simulink model "Test_World_1_cs"  (R2019a)
settings: Solver=FixedStepDiscrete  StartTime=0.0  StopTime=15  FixedStep=1/300  RelTol=1e-3
PreLoadFcn:
  | mbxruntime.callbacks.PreLoadFcn(bdroot);
  | check_NUTS_defined
  | model_closed = 0;
  | assignin('base',['model_closed_' bdroot],false);
PostLoadFcn:
  | mbxruntime.callbacks.PostLoadFcn(bdroot);
InitFcn:
  | mbxruntime.callbacks.InitFcn(bdroot);
StartFcn:
  | mbxruntime.callbacks.StartFcn(bdroot);
StopFcn:
  | mbxruntime.callbacks.StopFcn(bdroot);;
  | 
model workspace: external: MAT-File .\Test_World_1_cs_hws.mat (data not in the file)
undefined symbols (not defined in the file or in its folder): AngularVelocity, Clock_, Data, Data_SL_Info, DiscIntNeverNeededParam, Encoding, Encoding_SL_Info, Header, Height, InitImageOutputDir, LinearAcceleration, Orientation, Pose, Poses, Poses_SL_Info, Position, Step, Twist, Width
libraries: robotlib x26, simulink_extras x19, PreScanSimulinkLibrary x6, PBCSimulinkLibrary x5, dspindex x4, robotcorelib x2, sharedtransform x2, visionconversions x1, visionsinks x1
(part 3 of 5)

== system Test_World_1_cs/PointCloudSensor_3 ==
  Sensor : S-Function  FunctionName=sfun_PCS  Parameters=sensorID, dataWidth, dataHeight, numChannels, dataType, timestep  SFunctionDeploymentMode=off  EnableBusSupport=off  mask(PreScan Source Block: Point Cloud Sensor){sensorID=9054, dataWidth=16, dataHeight=900, numChannels=4, dataType=0, timestep=1/20}
      mask prompts: sensorID "Sensor ID"; dataWidth "Data Width"; dataHeight "Data Height"; numChannels "Channel Count"; dataType "Data Type"; timestep "MATLAB timestep:"
      mask help: The Point Cloud Sensor provides XYZ positions relative to the sensor
      mask Help: eval('openHelp(6400)')
      mask Display: image(imread('PointCloudSensorSL.png'))
  PointCloudSensor_3 : Outport  Tag=outport/PointCloudInport  OutDataTypeStr=single  SampleTime=1/20
  wires:
  Sensor/1 -> PointCloudSensor_3/1

== system Test_World_1_cs/PointCloudSensor_4 ==
  Sensor : S-Function  FunctionName=sfun_PCS  Parameters=sensorID, dataWidth, dataHeight, numChannels, dataType, timestep  SFunctionDeploymentMode=off  EnableBusSupport=off  mask(PreScan Source Block: Point Cloud Sensor){sensorID=9055, dataWidth=16, dataHeight=900, numChannels=4, dataType=0, timestep=1/20}
      mask prompts: sensorID "Sensor ID"; dataWidth "Data Width"; dataHeight "Data Height"; numChannels "Channel Count"; dataType "Data Type"; timestep "MATLAB timestep:"
      mask help: The Point Cloud Sensor provides XYZ positions relative to the sensor
      mask Help: eval('openHelp(6400)')
      mask Display: image(imread('PointCloudSensorSL.png'))
  PointCloudSensor_4 : Outport  Tag=outport/PointCloudInport  OutDataTypeStr=single  SampleTime=1/20
  wires:
  Sensor/1 -> PointCloudSensor_4/1

== system Test_World_1_cs/PreScanTerminator ==
  Terminator : Terminator
  sfun_Terminator : S-Function  FunctionName=sfun_Terminator  Parameters=SampleTime  SFunctionDeploymentMode=off  EnableBusSupport=off  mask(Legacy Function){SFunctionSpec=void prescan_terminator_outputFcn(void ** work1, PRESCAN_TERMINATORDATA y1[1]), SampleTime=TimeStep, ShowSpec=on}
      mask prompts: SampleTime "Sample time (-1 for inherited):"; ShowSpec "Display function specification"
      mask help:
      | This block allows you to call the legacy functions specified by the following Legacy Code Tool definition:
      | def.SFunctionName = 'sfun_Terminator';
      | def.OutputFcnSpec = 'void prescan_terminator_outputFcn(void ** work1, PRESCAN_TERMINATORDATA y1[1])';
      | def.StartFcnSpec = 'void prescan_terminator_startFcn(void ** work1)';
      | def.TerminateFcnSpec = 'void prescan_terminator_terminateFcn(void ** work1)';
      | def.HeaderFiles = {'prescan_terminator_data.h'};
      | def.HostLibFiles = {'sensorinterfaced.lib'};
      | def.IncPaths = {'src', 'C:\prescandev\vislibrary\vis\..\pimp\include\sensors\InterfaceRTW'};
      | def.SrcPaths = {'src'};
      | def.LibPaths = {'C:\\prescandev\\vislibrary_build\lib'};
      | def.SampleTime = 'parameterized';
      | def.Options.language = 'C';
      mask Help: <p>This block was generated automatically by the Legacy Code Tool. For detailed help on this tool, call<a href="matlab:legacy_code('help')"> legacy_code('help')</a>.</p>
      mask Callback ShowSpec:
      | if strcmp(get_param(gcbh, 'ShowSpec'), 'on')
      |   set_param(gcbh, 'MaskDisplay', sprintf('fprintf(''%s'');', get_param(gcbh, 'SFunctionSpec')));
      | else
      |   set_param(gcbh, 'MaskDisplay', sprintf('fprintf(''%s'');', get_param(gcbh, 'FunctionName')));
      | end
      mask Display: fprintf('void prescan_terminator_outputFcn(void ** work1, PRESCAN_TERMINATORDATA y1[1])');
  wires:
  sfun_Terminator/1 -> Terminator/1

== system Test_World_1_cs/SELF_BMW_X5_SUV_1 ==
  Sensor : S-Function  FunctionName=sfun_SelfSensor  Parameters=UniqueID, TimeStep  SFunctionDeploymentMode=off  EnableBusSupport=off  mask(PreScan Source Block: SELF){UniqueID=9040, TimeStep=1/300}
      mask prompts: UniqueID "Auto-Assigned: Unique ID"; TimeStep "Auto-Assigned: Upload Period [s]"
      mask help:
      | The SELF port shows (state) information of the actor itself. The outputs are position in the experiment's axis system and the GPS coordinates, and the object's absolute velocity and compass heading.
      |
      | For more information, please click Help.
      mask Help: eval('openHelp(462)')
      mask Display: image(imread('GPS.png'))
  SELF_BMW_X5_SUV_1 : Outport  Tag=outport/SelfPort  OutDataTypeStr=Bus: PRESCAN_SELFSENSORDATA  PortDimensions=1  SampleTime=1/300
  wires:
  Sensor/1 -> SELF_BMW_X5_SUV_1/1

== system Test_World_1_cs/SELF_Citroen_C3_Hatchback_1 ==
  Sensor : S-Function  FunctionName=sfun_SelfSensor  Parameters=UniqueID, TimeStep  SFunctionDeploymentMode=off  EnableBusSupport=off  mask(PreScan Source Block: SELF){UniqueID=4877, TimeStep=1/300}
      mask prompts: UniqueID "Auto-Assigned: Unique ID"; TimeStep "Auto-Assigned: Upload Period [s]"
      mask help:
      | The SELF port shows (state) information of the actor itself. The outputs are position in the experiment's axis system and the GPS coordinates, and the object's absolute velocity and compass heading.
      |
      | For more information, please click Help.
      mask Help: eval('openHelp(462)')
      mask Display: image(imread('GPS.png'))
  SELF_Citroen_C3_Hatchback_1 : Outport  Tag=outport/SelfPort  OutDataTypeStr=Bus: PRESCAN_SELFSENSORDATA  PortDimensions=1  SampleTime=1/300
  wires:
  Sensor/1 -> SELF_Citroen_C3_Hatchback_1/1

== system Test_World_1_cs/SELF_Ford_Fiesta_Hatchback_1 ==
  Sensor : S-Function  FunctionName=sfun_SelfSensor  Parameters=UniqueID, TimeStep  SFunctionDeploymentMode=off  EnableBusSupport=off  mask(PreScan Source Block: SELF){UniqueID=4876, TimeStep=1/300}
      mask prompts: UniqueID "Auto-Assigned: Unique ID"; TimeStep "Auto-Assigned: Upload Period [s]"
      mask help:
      | The SELF port shows (state) information of the actor itself. The outputs are position in the experiment's axis system and the GPS coordinates, and the object's absolute velocity and compass heading.
      |
      | For more information, please click Help.
      mask Help: eval('openHelp(462)')
      mask Display: image(imread('GPS.png'))
  SELF_Ford_Fiesta_Hatchback_1 : Outport  Tag=outport/SelfPort  OutDataTypeStr=Bus: PRESCAN_SELFSENSORDATA  PortDimensions=1  SampleTime=1/300
  wires:
  Sensor/1 -> SELF_Ford_Fiesta_Hatchback_1/1

== system Test_World_1_cs/STATE_BMW_X5_SUV_1_bus ==
  STATE_BMW_X5_SUV_1_bus : Inport  Tag=inport/StatePort  OutDataTypeStr=Bus: PRESCAN_STATEACTUATORDATA  PortDimensions=1  SampleTime=1/300  BusOutputAsStruct=on
  Actuator : S-Function  FunctionName=sfun_StateActuator  Parameters=UniqueID, TimeStep  SFunctionDeploymentMode=off  EnableBusSupport=off  mask(PreScan Sink Block: State){UniqueID=9040, TimeStep=1/300}
      mask prompts: UniqueID "Auto-Assigned: Unique ID"; TimeStep "Auto-Assigned: Upload Period [s]"
      mask help:
      | The Actor State contains a vector signal of size (9x1), containing the following signals:
      |
      | -  Position    	(x,y,z)             	[m]
      | -  Velocity    	(vx,vy,vz)         	[m/s]
      | -  Angles       	(Roll, Pitch, Yaw)	[rad]
      |
      | The Actor state is defined in the global axis system.
      | The state is superponed on the Initial position defined in the GUI.
      |
      | For more information, please click Help.
      mask Help: eval('openHelp(222)')
      mask Display: image(imread('State.png'))
  wires:
  STATE_BMW_X5_SUV_1_bus/1 -> Actuator/1

== system Test_World_1_cs/STATE_Citroen_C3_Hatchback_1_bus ==
  STATE_Citroen_C3_Hatchback_1_bus : Inport  Tag=inport/StatePort  OutDataTypeStr=Bus: PRESCAN_STATEACTUATORDATA  PortDimensions=1  SampleTime=1/300  BusOutputAsStruct=on
  Actuator : S-Function  FunctionName=sfun_StateActuator  Parameters=UniqueID, TimeStep  SFunctionDeploymentMode=off  EnableBusSupport=off  mask(PreScan Sink Block: State){UniqueID=4877, TimeStep=1/300}
      mask prompts: UniqueID "Auto-Assigned: Unique ID"; TimeStep "Auto-Assigned: Upload Period [s]"
      mask help:
      | The Actor State contains a vector signal of size (9x1), containing the following signals:
      |
      | -  Position    	(x,y,z)             	[m]
      | -  Velocity    	(vx,vy,vz)         	[m/s]
      | -  Angles       	(Roll, Pitch, Yaw)	[rad]
      |
      | The Actor state is defined in the global axis system.
      | The state is superponed on the Initial position defined in the GUI.
      |
      | For more information, please click Help.
      mask Help: eval('openHelp(222)')
      mask Display: image(imread('State.png'))
  wires:
  STATE_Citroen_C3_Hatchback_1_bus/1 -> Actuator/1

== system Test_World_1_cs/STATE_Ford_Fiesta_Hatchback_1_bus ==
  STATE_Ford_Fiesta_Hatchback_1_bus : Inport  Tag=inport/StatePort  OutDataTypeStr=Bus: PRESCAN_STATEACTUATORDATA  PortDimensions=1  SampleTime=1/300  BusOutputAsStruct=on
  Actuator : S-Function  FunctionName=sfun_StateActuator  Parameters=UniqueID, TimeStep  SFunctionDeploymentMode=off  EnableBusSupport=off  mask(PreScan Sink Block: State){UniqueID=4876, TimeStep=1/300}
      mask prompts: UniqueID "Auto-Assigned: Unique ID"; TimeStep "Auto-Assigned: Upload Period [s]"
      mask help:
      | The Actor State contains a vector signal of size (9x1), containing the following signals:
      |
      | -  Position    	(x,y,z)             	[m]
      | -  Velocity    	(vx,vy,vz)         	[m/s]
      | -  Angles       	(Roll, Pitch, Yaw)	[rad]
      |
      | The Actor state is defined in the global axis system.
      | The state is superponed on the Initial position defined in the GUI.
      |
      | For more information, please click Help.
      mask Help: eval('openHelp(222)')
      mask Display: image(imread('State.png'))
  wires:
  STATE_Ford_Fiesta_Hatchback_1_bus/1 -> Actuator/1

== system Test_World_1_cs/Synchronizer ==
  Bus Selector1 : BusSelector  OutputSignals=FederateStopped
  Stop Simulation : Stop
  sfun_Synchronizer : S-Function  FunctionName=sfun_Synchronizer  Parameters=SampleTime  SFunctionDeploymentMode=off  EnableBusSupport=off  mask(Legacy Function){SFunctionSpec=void prescan_synchronizer_outputFcn(void ** work1, PRESCAN_SYNCHRONIZEDATA y1[1]), SampleTime=TimeStep, ShowSpec=on}
      mask prompts: SampleTime "Sample time (-1 for inherited):"; ShowSpec "Display function specification"
      mask help:
      | This block allows you to call the legacy functions specified by the following Legacy Code Tool definition:
      | def.SFunctionName = 'sfun_Synchronizer';
      | def.OutputFcnSpec = 'void prescan_synchronizer_outputFcn(void ** work1, PRESCAN_SYNCHRONIZEDATA y1[1])';
      | def.StartFcnSpec = 'void prescan_synchronizer_startFcn(void ** work1)';
      | def.TerminateFcnSpec = 'void prescan_synchronizer_terminateFcn(void ** work1)';
      | def.HeaderFiles = {'prescan_synchronizer_data.h'};
      | def.HostLibFiles = {'sensorinterfaced.lib'};
      | def.IncPaths = {'src', 'C:\prescandev\vislibrary\vis\..\pimp\include\sensors\InterfaceRTW'};
      | def.SrcPaths = {'src'};
      | def.LibPaths = {'C:\\prescandev\\vislibrary_build\lib'};
      | def.SampleTime = 'parameterized';
      | def.Options.language = 'C';
      mask Help: <p>This block was generated automatically by the Legacy Code Tool. For detailed help on this tool, call<a href="matlab:legacy_code('help')"> legacy_code('help')</a>.</p>
      mask Callback ShowSpec:
      | if strcmp(get_param(gcbh, 'ShowSpec'), 'on')
      |   set_param(gcbh, 'MaskDisplay', sprintf('fprintf(''%s'');', get_param(gcbh, 'SFunctionSpec')));
      | else
      |   set_param(gcbh, 'MaskDisplay', sprintf('fprintf(''%s'');', get_param(gcbh, 'FunctionName')));
      | end
      mask Display: fprintf('void prescan_synchronizer_outputFcn(void ** work1, PRESCAN_SYNCHRONIZEDATA y1[1])');
  wires:
  Bus Selector1/1 -> Stop Simulation/1  "<FederateStopped>"
  sfun_Synchronizer/1 -> Bus Selector1/1

== system Test_World_1_cs/camera ==
  Sensor : S-Function  FunctionName=sfun_Camera  Parameters=sensorID, dataWidth, dataHeight, channelsPerImage, numberOfImages, timestep  SFunctionDeploymentMode=off  EnableBusSupport=off  mask(PreScan Source Block: Camera Sensor){sensorID=9056, dataWidth=720, dataHeight=2880, channelsPerImage=3, numberOfImages=1, timestep=1/20}
      mask prompts: sensorID "Sensor ID"; dataWidth "Data width"; dataHeight "Data Height"; channelsPerImage "Channels per image"; numberOfImages "Number of images"; timestep "MATLAB timestep:"
      mask help: The Camera Sensor provides a color or monochrome image.
      mask Help: eval('openHelp(457)')
      mask Display: image(imread('CameraSensor.png'))
  camera : Outport  Tag=outport/Camera/CameraSensor  OutDataTypeStr=uint8  SampleTime=1/20
  wires:
  Sensor/1 -> camera/1

== system Test_World_1_cs/pose_otheCar ==
  In1 : Inport
  Enable : EnablePort
  Add5 : Sum
  Assignment : Assignment  OutputInitialize=Specify size for each dimension in table  DiagnosticForDimensions=Warning  IndexOptions=Starting index (dialog)  Indices=1  OutputSizes=1
  Assignment2 : Assignment  OutputInitialize=Specify size for each dimension in table  DiagnosticForDimensions=Warning  IndexOptions=Starting index (dialog)  Indices=1  OutputSizes=1000
  Blank Message1 : robotlib/Blank Message  messageClass=Message  entityType=geometry_msgs/PoseArray  messageType=geometry_msgs/PoseArray  SampleTime=inf
      settings: SourceProductBaseCode=RO
  Bus Assignment3 : BusAssignment  AssignedSignals=Header.Seq,Header.FrameId,Header.FrameId_SL_Info.CurrentLength,Poses,Poses_SL_Info.CurrentLength
  Bus Selector : BusSelector  OutputSignals=Poses
  Bus Selector2 : BusSelector  OutputSignals=Header.FrameId
  Constant24 : Constant  OutDataTypeStr=uint32
  Constant25 : Constant  Value=uint8(['map'])
  Memory2 : Memory  InheritSampleTime=on
  Publish2 : robotlib/Publish  topicSource=Specify your own  topic=/pose_otherCar  messageType=geometry_msgs/PoseArray  messageQueueLength=1
      settings: SourceProductBaseCode=RO
  Width : Width  DataType=uint32
  Width5 : Width  DataType=uint32
  wires:
  Blank Message1/1 -> Bus Assignment3/1, Bus Selector2/1, Bus Selector/1
  Bus Selector2/1 -> Assignment2/1  "<FrameId>"
  Assignment2/1 -> Width5/1, Bus Assignment3/3
  Constant25/1 -> Assignment2/2
  Bus Assignment3/1 -> Publish2/1
  In1/1 -> Assignment/2
  Bus Selector/1 -> Assignment/1  "<Poses>"
  Width/1 -> Bus Assignment3/6
  Assignment/1 -> Width/1, Bus Assignment3/5
  Width5/1 -> Bus Assignment3/4
  Add5/1 -> Memory2/1, Bus Assignment3/2
  Memory2/1 -> Add5/1
  Constant24/1 -> Add5/2

== system Test_World_1_cs/tl_camera ==
  Sensor : S-Function  FunctionName=sfun_Camera  Parameters=sensorID, dataWidth, dataHeight, channelsPerImage, numberOfImages, timestep  SFunctionDeploymentMode=off  EnableBusSupport=off  mask(PreScan Source Block: Camera Sensor){sensorID=12017, dataWidth=720, dataHeight=2880, channelsPerImage=3, numberOfImages=1, timestep=1/20}
      mask prompts: sensorID "Sensor ID"; dataWidth "Data width"; dataHeight "Data Height"; channelsPerImage "Channels per image"; numberOfImages "Number of images"; timestep "MATLAB timestep:"
      mask help: The Camera Sensor provides a color or monochrome image.
      mask Help: eval('openHelp(457)')
      mask Display: image(imread('CameraSensor.png'))
  tl_camera : Outport  Tag=outport/Camera/CameraSensor  OutDataTypeStr=uint8  SampleTime=1/20
  wires:
  Sensor/1 -> tl_camera/1

== system Test_World_1_cs/BMW_X5_SUV_1/Car_Pose ==
  In1 : Inport
  In2 : Inport  Port=2
  In3 : Inport  Port=3
  In4 : Inport  Port=4
  In5 : Inport  Port=5
  In6 : Inport  Port=6
  Coordinate Transformation Conversion : robotcorelib/Coordinate Transformation Conversion  InputRepresentation=Euler Angles  InputEulerSequence=XYZ  ShowTrVecInputPort=on  OutputRepresentation=Quaternion  OutputEulerSequence=ZYX  ShowTrVecOutputPort=on  SimulateUsing=Interpreted execution
      settings: SourceProductBaseCode=RO
  Data Type Conversion : DataTypeConversion
  Data Type Conversion1 : DataTypeConversion
  Data Type Conversion2 : DataTypeConversion
  Degrees to Radians1 : simulink_extras/Transformations/Degrees to Radians
  Degrees to Radians2 : simulink_extras/Transformations/Degrees to Radians
  Degrees to Radians5 : simulink_extras/Transformations/Degrees to Radians
  Mux : Mux
  Vector Concatenate2 : Concatenate  NumInputs=3
  Out1 : Outport
  wires:
  Degrees to Radians1/1 -> Vector Concatenate2/2
  Degrees to Radians5/1 -> Vector Concatenate2/1
  Vector Concatenate2/1 -> Coordinate Transformation Conversion/1
  Degrees to Radians2/1 -> Vector Concatenate2/3
  In1/1 -> Data Type Conversion/1
  In2/1 -> Data Type Conversion1/1
  In3/1 -> Data Type Conversion2/1
  In4/1 -> Degrees to Radians5/1
  In5/1 -> Degrees to Radians1/1
  In6/1 -> Degrees to Radians2/1
  Data Type Conversion/1 -> Mux/1
  Data Type Conversion1/1 -> Mux/2
  Data Type Conversion2/1 -> Mux/3
  Coordinate Transformation Conversion/1 -> Mux/4
  Mux/1 -> Out1/1

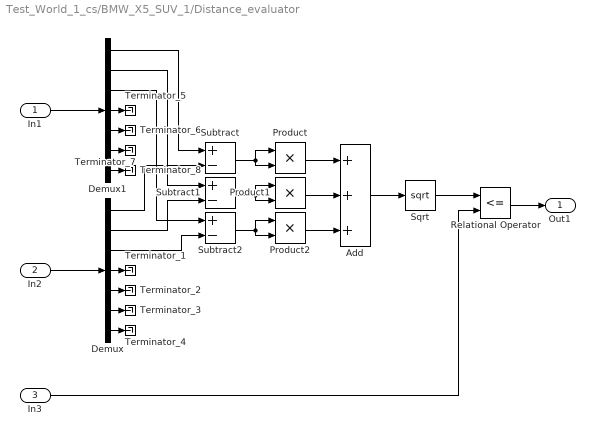
== system Test_World_1_cs/BMW_X5_SUV_1/Distance_evaluator ==
  In1 : Inport
  In2 : Inport  Port=2
  In3 : Inport  Port=3
  Add : Sum  Inputs=3
  Demux : Demux  Outputs=7
  Demux1 : Demux  Outputs=7
  Product : Product
  Product1 : Product
  Product2 : Product
  Relational Operator : RelationalOperator  Operator=<=  OutDataTypeStr=boolean  RndMeth=Simplest
  Sqrt : Sqrt  SaturateOnIntegerOverflow=on
  Subtract : Sum  Inputs=+-
  Subtract1 : Sum  Inputs=+-
  Subtract2 : Sum  Inputs=+-
  Terminator_{1..8} (8 alike) : Terminator
  Out1 : Outport
  wires:
  Relational Operator/1 -> Out1/1
  In1/1 -> Demux1/1
  In2/1 -> Demux/1
  Demux1/1 -> Subtract/1
  Demux1/2 -> Subtract1/1
  Demux1/3 -> Subtract2/1
  Demux/1 -> Subtract/2
  Demux/2 -> Subtract1/2
  Demux/3 -> Subtract2/2
  Subtract/1 -> Product/1, Product/2
  Subtract1/1 -> Product1/1, Product1/2
  Subtract2/1 -> Product2/1, Product2/2
  Product/1 -> Add/1
  Product1/1 -> Add/2
  Product2/1 -> Add/3
  Add/1 -> Sqrt/1
  Sqrt/1 -> Relational Operator/1
  In3/1 -> Relational Operator/2
  Demux/4 -> Terminator_1/1
  Demux/5 -> Terminator_2/1
  Demux/6 -> Terminator_3/1
  Demux/7 -> Terminator_4/1
  Demux1/4 -> Terminator_5/1
  Demux1/5 -> Terminator_6/1
  Demux1/6 -> Terminator_7/1
  Demux1/7 -> Terminator_8/1

== system Test_World_1_cs/BMW_X5_SUV_1/Dynamics_Empty ==
  note: For state mode 'Dynamic' positions
      | are not taken into account, as they
      | are computed by integrating velocity.
      | Click annotation for Help.
  Bus Selector : BusSelector  OutputSignals=Twist.Linear.X,Twist.Linear.Y,Twist.Linear.Z,Twist.Angular.X,Twist.Angular.Y,Twist.Angular.Z
  Data Type Conversion{,1..5} (6 alike) : DataTypeConversion
  Discrete-Time Integrator1 : DiscreteIntegrator  SampleTime=-1  ICPrevOutput=DiscIntNeverNeededParam  ICPrevScaledInput=DiscIntNeverNeededParam
  Discrete-Time Integrator2 : DiscreteIntegrator  SampleTime=-1  ICPrevOutput=DiscIntNeverNeededParam  ICPrevScaledInput=DiscIntNeverNeededParam
  Discrete-Time Integrator3 : DiscreteIntegrator  SampleTime=-1  ICPrevOutput=DiscIntNeverNeededParam  ICPrevScaledInput=DiscIntNeverNeededParam
  Ground_1 : Ground
  Ground_2 : Ground
  Ground_3 : Ground
  MuxState : Subsystem  Tag=mux/State  mask(Empty Dynamics State Block){positioningmode=off, TimeStep=1/300}
      mask prompts: positioningmode "Positioning Mode"; TimeStep "Auto Assigned: Time Step [s]"
      mask help:
      | Build the state of an actor based on user input.
      | The user can either use positioning mode or dynamics mode.
      | - When using positioning mode the position and orientation of the actor are set directly based on the input. Expected input is relative to the initial position and orientation of the actor. It's also possible to specify the velocity of the actor, though this input isn't used, only passed on.
      | - When using dynamics mode the position input is ignored. Expected input is velocity and orientation. The velocity is relative the current orientation of the actor, while orientation is relative to its initial orientation. The position of the actor is calculated based on the velocity and orientation given.
      settings: DeleteFcn=PreScanBlockDeleteFcn;
  STATE_BMW_X5_SUV_1 : Subsystem  Tag=mux/StatePort  Priority=0  LoadFcn=load PrescanStateActuatorData  mask(PreScan Sink Block: State){x0=19.2335, y0=197.6423, z0=0.69, Roll0=0, Pitch0=0, Yaw0=0.26655, TimeStep=1/300}
      mask prompts: x0 "Ini x-position VEHICLE wrt GLOBAL axis system [m]"; y0 "Ini y-position VEHICLE wrt GLOBAL axis system [m]"; z0 "Ini z-position VEHICLE wrt GLOBAL axis system [m]"; Roll0 "Ini roll-angle BODY wrt VEHICLE axis system [deg]"; Pitch0 "Ini pitch-angle BODY wrt VEHICLE axis system [deg]"; Yaw0 "Ini yaw-angle VEHICLE wrt GLOBAL axis system [deg]"; TimeStep "Auto-Assigned: Upload Period [s]"
      mask help:
      | The Actor State contains a vector signal of size (9x1), containing the following signals:
      |
      | -  Position                  (x,y,z)                                     [m]
      | -  Velocity                  (vx,vy,vz)                               [m/s]
      | -  Angles                    (Roll, Pitch, Yaw)                   [rad]
      |
      | The Actor state is defined in the global axis system.
      | The state is superponed on the Initial position defined in the GUI.
      |
      | For more information, please click Help.
      settings: DeleteFcn=PreScanBlockDeleteFcn;
      mask Help: eval('openHelp(222)')
      mask Display: image(imread('State.png'))
  Scope : Scope
  Sine Wave Function : Sin  Amplitude=0.1  SampleTime=0
  Subscribe : robotlib/Subscribe  topicSource=Select from ROS network  topic=/TwistS  messageType=geometry_msgs/TwistStamped  sampleTime=-1  messageQueueLength=1
      settings: SourceProductBaseCode=RO
  Terminator_1 : Terminator
  Terminator_2 : Terminator
  State : Outport  Tag=outport/StateOutport  SampleTime=1/300
  tag scope: x_speed=global
  wires:
  Bus Selector/1 -> Data Type Conversion/1, Scope/1  "<X>"
  Bus Selector/2 -> Data Type Conversion1/1  "<Y>"
  Bus Selector/3 -> Data Type Conversion2/1  "<Z>"
  Bus Selector/4 -> Data Type Conversion3/1  "<X>"
  Data Type Conversion3/1 -> Discrete-Time Integrator3/1
  Bus Selector/5 -> Data Type Conversion4/1  "<Y>"
  Data Type Conversion4/1 -> Discrete-Time Integrator2/1
  Bus Selector/6 -> Data Type Conversion5/1  "<Z>"
  Data Type Conversion5/1 -> Discrete-Time Integrator1/1
  Subscribe/2 -> Bus Selector/1
  Data Type Conversion/1 -> [x_speed], MuxState/4(dx [m/s])
  Data Type Conversion1/1 -> MuxState/5(dy [m/s])
  Data Type Conversion2/1 -> MuxState/6(dz [m/s])
  Discrete-Time Integrator3/1 -> MuxState/7(R [rad])
  Discrete-Time Integrator2/1 -> MuxState/8(P [rad])
  Discrete-Time Integrator1/1 -> MuxState/9(Y [rad])
  MuxState/1(state) -> STATE_BMW_X5_SUV_1/1(State)
  STATE_BMW_X5_SUV_1/1(StateBus) -> State/1
  Ground_1/1 -> MuxState/1(x [m])
  Ground_2/1 -> MuxState/2(y [m])
  Ground_3/1 -> MuxState/3(z [m])
  Sine Wave Function/1 -> Terminator_1/1
  Subscribe/1 -> Terminator_2/1

== system Test_World_1_cs/BMW_X5_SUV_1/Frequency evaluator ==
  In1 : Inport
  Add : Sum  Inputs=+-
  Clock2 : Clock
  Constant : Constant
  Divide : Product  Inputs=*/
  Memory : Memory
  Relational Operator : RelationalOperator  OutDataTypeStr=boolean  RndMeth=Simplest
  Switch : Switch  Criteria=u2 > Threshold
  Out1 : Outport
  wires:
  Memory/1 -> Switch/3, Add/2
  Switch/1 -> Memory/1
  Add/1 -> Relational Operator/1
  Relational Operator/1 -> Switch/2, Out1/1
  Clock2/1 -> Add/1, Switch/1
  In1/1 -> Divide/2
  Constant/1 -> Divide/1
  Divide/1 -> Relational Operator/2

== system Test_World_1_cs/BMW_X5_SUV_1/Frequency evaluator1 ==
  In1 : Inport
  Add : Sum  Inputs=+-
  Clock2 : Clock
  Constant : Constant
  Divide : Product  Inputs=*/
  Memory : Memory
  Relational Operator : RelationalOperator  OutDataTypeStr=boolean  RndMeth=Simplest
  Switch : Switch  Criteria=u2 > Threshold
  Out1 : Outport
  wires:
  Memory/1 -> Switch/3, Add/2
  Switch/1 -> Memory/1
  Add/1 -> Relational Operator/1
  Relational Operator/1 -> Switch/2, Out1/1
  Clock2/1 -> Add/1, Switch/1
  In1/1 -> Divide/2
  Constant/1 -> Divide/1
  Divide/1 -> Relational Operator/2

== system Test_World_1_cs/BMW_X5_SUV_1/Frequency evaluator2 ==
  In1 : Inport
  Add : Sum  Inputs=+-
  Clock2 : Clock
  Constant : Constant
  Divide : Product  Inputs=*/
  Memory : Memory
  Relational Operator : RelationalOperator  OutDataTypeStr=boolean  RndMeth=Simplest
  Switch : Switch  Criteria=u2 > Threshold
  Out1 : Outport
  wires:
  Memory/1 -> Switch/3, Add/2
  Switch/1 -> Memory/1
  Add/1 -> Relational Operator/1
  Relational Operator/1 -> Switch/2, Out1/1
  Clock2/1 -> Add/1, Switch/1
  In1/1 -> Divide/2
  Constant/1 -> Divide/1
  Divide/1 -> Relational Operator/2

== system Test_World_1_cs/BMW_X5_SUV_1/Frequency evaluator3 ==
  In1 : Inport
  Add : Sum  Inputs=+-
  Clock2 : Clock
  Constant : Constant
  Divide : Product  Inputs=*/
  Memory : Memory
  Relational Operator : RelationalOperator  OutDataTypeStr=boolean  RndMeth=Simplest
  Switch : Switch  Criteria=u2 > Threshold
  Out1 : Outport
  wires:
  Memory/1 -> Switch/3, Add/2
  Switch/1 -> Memory/1
  Add/1 -> Relational Operator/1
  Relational Operator/1 -> Switch/2, Out1/1
  Clock2/1 -> Add/1, Switch/1
  In1/1 -> Divide/2
  Constant/1 -> Divide/1
  Divide/1 -> Relational Operator/2

== system Test_World_1_cs/BMW_X5_SUV_1/Frequency evaluator4 ==
  In1 : Inport
  Add : Sum  Inputs=+-
  Clock2 : Clock
  Constant : Constant
  Divide : Product  Inputs=*/
  Memory : Memory
  Relational Operator : RelationalOperator  OutDataTypeStr=boolean  RndMeth=Simplest
  Switch : Switch  Criteria=u2 > Threshold
  Out1 : Outport
  wires:
  Memory/1 -> Switch/3, Add/2
  Switch/1 -> Memory/1
  Add/1 -> Relational Operator/1
  Relational Operator/1 -> Switch/2, Out1/1
  Clock2/1 -> Add/1, Switch/1
  In1/1 -> Divide/2
  Constant/1 -> Divide/1
  Divide/1 -> Relational Operator/2

== system Test_World_1_cs/BMW_X5_SUV_1/Frequency evaluator5 ==
  In1 : Inport
  Add : Sum  Inputs=+-
  Clock2 : Clock
  Constant : Constant
  Divide : Product  Inputs=*/
  Memory : Memory
  Relational Operator : RelationalOperator  OutDataTypeStr=boolean  RndMeth=Simplest
  Switch : Switch  Criteria=u2 > Threshold
  Out1 : Outport
  wires:
  Memory/1 -> Switch/3, Add/2
  Switch/1 -> Memory/1
  Add/1 -> Relational Operator/1
  Relational Operator/1 -> Switch/2, Out1/1
  Clock2/1 -> Add/1, Switch/1
  In1/1 -> Divide/2
  Constant/1 -> Divide/1
  Divide/1 -> Relational Operator/2

== system Test_World_1_cs/BMW_X5_SUV_1/Frequency evaluator6 ==
  In1 : Inport
  Add : Sum  Inputs=+-
  Clock2 : Clock
  Constant : Constant
  Divide : Product  Inputs=*/
  Memory : Memory
  Relational Operator : RelationalOperator  OutDataTypeStr=boolean  RndMeth=Simplest
  Switch : Switch  Criteria=u2 > Threshold
  Out1 : Outport
  wires:
  Divide/1 -> Relational Operator/2
  Constant/1 -> Divide/1
  In1/1 -> Divide/2
  Clock2/1 -> Switch/1, Add/1
  Relational Operator/1 -> Out1/1, Switch/2
  Add/1 -> Relational Operator/1
  Switch/1 -> Memory/1
  Memory/1 -> Add/2, Switch/3

== system Test_World_1_cs/BMW_X5_SUV_1/Frequency evaluator7 ==
  In1 : Inport
  Add : Sum  Inputs=+-
  Clock2 : Clock
  Constant : Constant
  Divide : Product  Inputs=*/
  Memory : Memory
  Relational Operator : RelationalOperator  OutDataTypeStr=boolean  RndMeth=Simplest
  Switch : Switch  Criteria=u2 > Threshold
  Out1 : Outport
  wires:
  Divide/1 -> Relational Operator/2
  Constant/1 -> Divide/1
  In1/1 -> Divide/2
  Clock2/1 -> Switch/1, Add/1
  Relational Operator/1 -> Out1/1, Switch/2
  Add/1 -> Relational Operator/1
  Switch/1 -> Memory/1
  Memory/1 -> Add/2, Switch/3

== system Test_World_1_cs/BMW_X5_SUV_1/HumViewCamera_CM_Demux ==
  In1 : Inport
  Selector : Selector  NumberOfDimensions=2  InputPortWidth=3  IndexOptions=Index vector (dialog),Index vector (dialog)  Indices=-1,1:hres  OutputSizes=1,1
  Selector1 : Selector  NumberOfDimensions=2  InputPortWidth=3  IndexOptions=Index vector (dialog),Index vector (dialog)  Indices=-1,hres+1:hres*2  OutputSizes=1,1
  Selector2 : Selector  NumberOfDimensions=2  InputPortWidth=3  IndexOptions=Index vector (dialog),Index vector (dialog)  Indices=-1,hres*2+1:hres*3  OutputSizes=1,1
  R : Outport
  G : Outport  Port=2
  B : Outport  Port=3
  wires:
  In1/1 -> Selector1/1, Selector/1, Selector2/1
  Selector/1 -> R/1
  Selector1/1 -> G/1
  Selector2/1 -> B/1

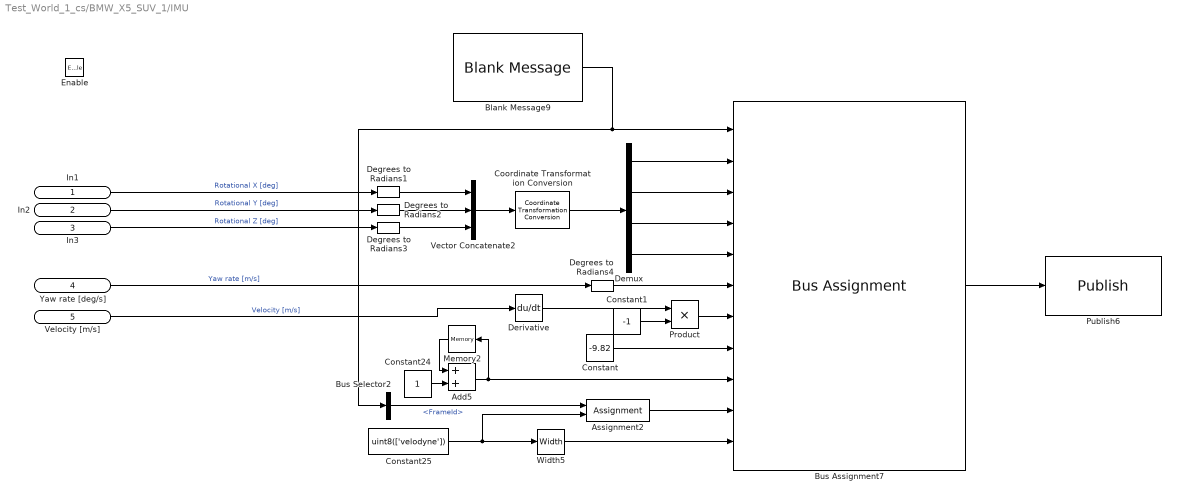
== system Test_World_1_cs/BMW_X5_SUV_1/IMU ==
  In1 : Inport
  In2 : Inport  Port=2
  In3 : Inport  Port=3
  Yaw rate [deg/s] : Inport  Port=4
  Velocity [m/s] : Inport  Port=5
  Enable : EnablePort
  Add5 : Sum
  Assignment2 : Assignment  OutputInitialize=Specify size for each dimension in table  DiagnosticForDimensions=Warning  IndexOptions=Starting index (dialog)  Indices=1  OutputSizes=1000
  Blank Message9 : robotlib/Blank Message  messageClass=Message  entityType=sensor_msgs/Imu  messageType=sensor_msgs/Imu  SampleTime=inf
      settings: SourceProductBaseCode=RO
  Bus Assignment7 : BusAssignment  AssignedSignals=Orientation.W,Orientation.X,Orientation.Y,Orientation.Z,AngularVelocity.Z,LinearAcceleration.X,LinearAcceleration.Z,Header.Seq,Header.FrameId,Header.FrameId_SL_Info.CurrentLength
  Bus Selector2 : BusSelector  OutputSignals=Header.FrameId
  Constant : Constant  Value=-9.82
  Constant1 : Constant  Value=-1
  Constant24 : Constant  OutDataTypeStr=uint32
  Constant25 : Constant  Value=uint8(['velodyne'])
  Coordinate Transformation Conversion : robotcorelib/Coordinate Transformation Conversion  InputRepresentation=Euler Angles  InputEulerSequence=XYZ  ShowTrVecInputPort=on  OutputRepresentation=Quaternion  OutputEulerSequence=ZYX  ShowTrVecOutputPort=on  SimulateUsing=Interpreted execution
      settings: SourceProductBaseCode=RO
  Degrees to Radians{1..4} (4 alike) : simulink_extras/Transformations/Degrees to Radians
  Demux : Demux
  Derivative : Derivative
  Memory2 : Memory  InheritSampleTime=on
  Product : Product
  Publish6 : robotlib/Publish  topicSource=Select from ROS network  topic=/imu_raw  messageType=sensor_msgs/Imu  messageQueueLength=1
      settings: SourceProductBaseCode=RO
  Vector Concatenate2 : Concatenate  NumInputs=3
  Width5 : Width  DataType=uint32
  wires:
  Product/1 -> Bus Assignment7/7
  Constant1/1 -> Product/2
  In3/1 -> Degrees to Radians3/1  "Rotational Z [deg]"
  In2/1 -> Degrees to Radians2/1  "Rotational Y [deg]"
  In1/1 -> Degrees to Radians1/1  "Rotational X [deg]"
  Constant/1 -> Bus Assignment7/8
  Velocity [m/s]/1 -> Derivative/1  "Velocity [m/s]"
  Yaw rate [deg/s]/1 -> Degrees to Radians4/1  "Yaw rate [m/s]"
  Demux/4 -> Bus Assignment7/5
  Demux/1 -> Bus Assignment7/2
  Coordinate Transformation Conversion/1 -> Demux/1
  Demux/3 -> Bus Assignment7/4
  Vector Concatenate2/1 -> Coordinate Transformation Conversion/1
  Degrees to Radians3/1 -> Vector Concatenate2/3
  Demux/2 -> Bus Assignment7/3
  Degrees to Radians2/1 -> Vector Concatenate2/2
  Derivative/1 -> Product/1
  Assignment2/1 -> Bus Assignment7/10
  Degrees to Radians4/1 -> Bus Assignment7/6
  Memory2/1 -> Add5/1
  Bus Assignment7/1 -> Publish6/1
  Add5/1 -> Bus Assignment7/9, Memory2/1
  Width5/1 -> Bus Assignment7/11
  Blank Message9/1 -> Bus Assignment7/1, Bus Selector2/1
  Bus Selector2/1 -> Assignment2/1  "<FrameId>"
  Constant25/1 -> Width5/1, Assignment2/2
  Constant24/1 -> Add5/2
  Degrees to Radians1/1 -> Vector Concatenate2/1

== system Test_World_1_cs/BMW_X5_SUV_1/PhysicsBasedCameraSensor_1_PBCPose_Control_Mux ==
  Position [m] : Inport
  Orientation [rad] : Inport  Port=2
  Bus Creator1 : BusCreator  Inputs=12  OutDataTypeStr=Bus: PRESCAN_PBCPOSE_DATA  NonVirtualBus=on
  Demux{,1..3} (4 alike) : Demux  Outputs=3
  SignalChanged : PBCSimulinkLibrary/SignalChanged  SystemSampleTime=-1
  SignalChanged1 : PBCSimulinkLibrary/SignalChanged  SystemSampleTime=-1
  Bus : Outport
  wires:
  Demux1/3 -> Bus Creator1/12  "OrientationYaw"
  Demux1/2 -> Bus Creator1/11  "OrientationPitch"
  Demux1/1 -> Bus Creator1/10  "OrientationRoll"
  Demux3/3 -> Bus Creator1/9  "OrientationYawDefined"
  Demux3/2 -> Bus Creator1/8  "OrientationPitchDefined"
  Demux3/1 -> Bus Creator1/7  "OrientationRollDefined"
  Demux/3 -> Bus Creator1/6  "PositionZ"
  Demux/2 -> Bus Creator1/5  "PositionY"
  Demux/1 -> Bus Creator1/4  "PositionX"
  Demux2/3 -> Bus Creator1/3  "PositionZDefined"
  Demux2/2 -> Bus Creator1/2  "PositionYDefined"
  Demux2/1 -> Bus Creator1/1  "PositionXDefined"
  SignalChanged1/1 -> Demux3/1
  SignalChanged/1 -> Demux2/1
  Bus Creator1/1 -> Bus/1
  Position [m]/1 -> SignalChanged/1, Demux/1
  Orientation [rad]/1 -> SignalChanged1/1, Demux1/1

== system Test_World_1_cs/BMW_X5_SUV_1/PhysicsBasedCameraSensor_1_PBC_Control_Mux ==
  IntegrationTime [s] : Inport
  DigitalGain [-] : Inport  Port=2
  InterRowIntegrationDelay [s] : Inport  Port=3
  AnalogGain : Constant  Value=0
  AnalogGainDefined : Constant  Value=false
  Bus Creator1 : BusCreator  Inputs=14  OutDataTypeStr=Bus: PRESCAN_PBCCONTROL_DATA  NonVirtualBus=on
  DigitalGain1 : Constant  Value=0
  DigitalGain2 : Constant  Value=0
  DigitalGain3 : Constant  Value=0
  DigitalGainDefined1 : Constant  Value=false
  DigitalGainDefined2 : Constant  Value=false
  DigitalGainDefined3 : Constant  Value=false
  NonNegativeSignalChanged1 : PBCSimulinkLibrary/NonNegativeSignalChanged  SystemSampleTime=-1
  NonNegativeSignalChanged2 : PBCSimulinkLibrary/NonNegativeSignalChanged  SystemSampleTime=-1
  NonNegativeSignalChanged7 : PBCSimulinkLibrary/NonNegativeSignalChanged  SystemSampleTime=-1
  Bus : Outport
  wires:
  NonNegativeSignalChanged7/1 -> Bus Creator1/13  "InterRowIntegrationDelayDefined"
  InterRowIntegrationDelay [s]/1 -> Bus Creator1/14, NonNegativeSignalChanged7/1  "InterRowIntegrationDelay"
  AnalogGainDefined/1 -> Bus Creator1/11  "AnalogGainDefined"
  AnalogGain/1 -> Bus Creator1/12  "AnalogGain"
  DigitalGainDefined3/1 -> Bus Creator1/9  "DigitalGain3Defined"
  DigitalGainDefined2/1 -> Bus Creator1/7  "DigitalGain2Defined"
  DigitalGainDefined1/1 -> Bus Creator1/5  "DigitalGain1Defined"
  NonNegativeSignalChanged2/1 -> Bus Creator1/3  "DigitalGain0Defined"
  NonNegativeSignalChanged1/1 -> Bus Creator1/1  "IntegrationTimeDefined"
  DigitalGain3/1 -> Bus Creator1/10  "DigitalGain3"
  DigitalGain2/1 -> Bus Creator1/8  "DigitalGain2"
  DigitalGain1/1 -> Bus Creator1/6  "DigitalGain1"
  DigitalGain [-]/1 -> Bus Creator1/4, NonNegativeSignalChanged2/1  "DigitalGain0"
  IntegrationTime [s]/1 -> Bus Creator1/2, NonNegativeSignalChanged1/1  "IntegrationTime"
  Bus Creator1/1 -> Bus/1

== system Test_World_1_cs/BMW_X5_SUV_1/PhysicsBasedCameraSensor_1_capture_opticsandsensor_Demux ==
  note: This block exists for legacy compatibility only
  In1 : Inport
  I : Outport
  wires:
  In1/1 -> I/1

== system Test_World_1_cs/BMW_X5_SUV_1/PointCloudSensor_1_Angles_Demux ==
  In2 : Inport
  Selector : Selector  NumberOfDimensions=2  InputPortWidth=3  IndexOptions=Index vector (dialog),Index vector (dialog)  Indices=-1,offset+1:(offset+hres)  OutputSizes=1,1
  Selector1 : Selector  NumberOfDimensions=2  InputPortWidth=3  IndexOptions=Index vector (dialog),Index vector (dialog)  Indices=-1,(offset+hres+1):(offset+2*hres)  OutputSizes=1,1
  Theta : Outport
  Phi : Outport  Port=2
  wires:
  Selector1/1 -> Phi/1
  Selector/1 -> Theta/1
  In2/1 -> Selector/1, Selector1/1

== system Test_World_1_cs/BMW_X5_SUV_1/PointCloudSensor_1_Intensity_Demux ==
  In1 : Inport
  Selector3 : Selector  NumberOfDimensions=2  InputPortWidth=3  IndexOptions=Index vector (dialog),Index vector (dialog)  Indices=-1,offset+1:(offset+hres)  OutputSizes=1,1
  Intensity : Outport
  wires:
  Selector3/1 -> Intensity/1
  In1/1 -> Selector3/1

== system Test_World_1_cs/BMW_X5_SUV_1/PointCloudSensor_1_Range_Demux ==
  In1 : Inport
  Selector : Selector  NumberOfDimensions=2  InputPortWidth=3  IndexOptions=Index vector (dialog),Index vector (dialog)  Indices=-1,offset+1:(offset+hres)  OutputSizes=1,1
  Range : Outport
  wires:
  Selector/1 -> Range/1
  In1/1 -> Selector/1

== system Test_World_1_cs/BMW_X5_SUV_1/PointCloudSensor_2_Angles_Demux ==
  In2 : Inport
  Selector : Selector  NumberOfDimensions=2  InputPortWidth=3  IndexOptions=Index vector (dialog),Index vector (dialog)  Indices=-1,offset+1:(offset+hres)  OutputSizes=1,1
  Selector1 : Selector  NumberOfDimensions=2  InputPortWidth=3  IndexOptions=Index vector (dialog),Index vector (dialog)  Indices=-1,(offset+hres+1):(offset+2*hres)  OutputSizes=1,1
  Theta : Outport
  Phi : Outport  Port=2
  wires:
  Selector1/1 -> Phi/1
  Selector/1 -> Theta/1
  In2/1 -> Selector/1, Selector1/1

== system Test_World_1_cs/BMW_X5_SUV_1/PointCloudSensor_2_Intensity_Demux ==
  In1 : Inport
  Selector3 : Selector  NumberOfDimensions=2  InputPortWidth=3  IndexOptions=Index vector (dialog),Index vector (dialog)  Indices=-1,offset+1:(offset+hres)  OutputSizes=1,1
  Intensity : Outport
  wires:
  Selector3/1 -> Intensity/1
  In1/1 -> Selector3/1

== system Test_World_1_cs/BMW_X5_SUV_1/PointCloudSensor_2_Range_Demux ==
  In1 : Inport
  Selector : Selector  NumberOfDimensions=2  InputPortWidth=3  IndexOptions=Index vector (dialog),Index vector (dialog)  Indices=-1,offset+1:(offset+hres)  OutputSizes=1,1
  Range : Outport
  wires:
  Selector/1 -> Range/1
  In1/1 -> Selector/1

== system Test_World_1_cs/BMW_X5_SUV_1/PointCloudSensor_3_Angles_Demux ==
  In2 : Inport
  Selector : Selector  NumberOfDimensions=2  InputPortWidth=3  IndexOptions=Index vector (dialog),Index vector (dialog)  Indices=-1,offset+1:(offset+hres)  OutputSizes=1,1
  Selector1 : Selector  NumberOfDimensions=2  InputPortWidth=3  IndexOptions=Index vector (dialog),Index vector (dialog)  Indices=-1,(offset+hres+1):(offset+2*hres)  OutputSizes=1,1
  Theta : Outport
  Phi : Outport  Port=2
  wires:
  Selector1/1 -> Phi/1
  Selector/1 -> Theta/1
  In2/1 -> Selector/1, Selector1/1

== system Test_World_1_cs/BMW_X5_SUV_1/PointCloudSensor_3_Intensity_Demux ==
  In1 : Inport
  Selector3 : Selector  NumberOfDimensions=2  InputPortWidth=3  IndexOptions=Index vector (dialog),Index vector (dialog)  Indices=-1,offset+1:(offset+hres)  OutputSizes=1,1
  Intensity : Outport
  wires:
  Selector3/1 -> Intensity/1
  In1/1 -> Selector3/1

== system Test_World_1_cs/BMW_X5_SUV_1/PointCloudSensor_3_Range_Demux ==
  In1 : Inport
  Selector : Selector  NumberOfDimensions=2  InputPortWidth=3  IndexOptions=Index vector (dialog),Index vector (dialog)  Indices=-1,offset+1:(offset+hres)  OutputSizes=1,1
  Range : Outport
  wires:
  Selector/1 -> Range/1
  In1/1 -> Selector/1

== system Test_World_1_cs/BMW_X5_SUV_1/PointCloudSensor_4_Angles_Demux ==
  In2 : Inport
  Selector : Selector  NumberOfDimensions=2  InputPortWidth=3  IndexOptions=Index vector (dialog),Index vector (dialog)  Indices=-1,offset+1:(offset+hres)  OutputSizes=1,1
  Selector1 : Selector  NumberOfDimensions=2  InputPortWidth=3  IndexOptions=Index vector (dialog),Index vector (dialog)  Indices=-1,(offset+hres+1):(offset+2*hres)  OutputSizes=1,1
  Theta : Outport
  Phi : Outport  Port=2
  wires:
  Selector1/1 -> Phi/1
  Selector/1 -> Theta/1
  In2/1 -> Selector/1, Selector1/1

== system Test_World_1_cs/BMW_X5_SUV_1/PointCloudSensor_4_Intensity_Demux ==
  In1 : Inport
  Selector3 : Selector  NumberOfDimensions=2  InputPortWidth=3  IndexOptions=Index vector (dialog),Index vector (dialog)  Indices=-1,offset+1:(offset+hres)  OutputSizes=1,1
  Intensity : Outport
  wires:
  Selector3/1 -> Intensity/1
  In1/1 -> Selector3/1

== system Test_World_1_cs/BMW_X5_SUV_1/PointCloudSensor_4_Range_Demux ==
  In1 : Inport
  Selector : Selector  NumberOfDimensions=2  InputPortWidth=3  IndexOptions=Index vector (dialog),Index vector (dialog)  Indices=-1,offset+1:(offset+hres)  OutputSizes=1,1
  Range : Outport
  wires:
  Selector/1 -> Range/1
  In1/1 -> Selector/1

== system Test_World_1_cs/BMW_X5_SUV_1/SELF_Demux ==
  SELF : Inport  OutDataTypeStr=Bus: PRESCAN_SELFSENSORDATA
  Bus Selector : BusSelector  OutputSignals=PositionX,PositionY,PositionZ,OrientationRoll,OrientationPitch,OrientationYaw,Velocity,Yaw_rate,Lat,Long,Alt
  Demux2 : Demux  Outputs=3
  Gain : Gain  Gain=180/pi
  Gain1 : Gain  Gain=180/pi
  Vector Concatenate1 : Concatenate  NumInputs=3
  compas converter : Subsystem
  x [m] : Outport
  y [m] : Outport  Port=2
  z [m] : Outport  Port=3
  rotx [deg] : Outport  Port=4
  roty [deg] : Outport  Port=5
  rotz [deg] : Outport  Port=6
  GPS lat [deg] : Outport  Port=7
  GPS long [deg] : Outport  Port=8
  GPS alt [m] : Outport  Port=9
  velocity [m/s] : Outport  Port=10
  heading [deg] : Outport  Port=11
  yaw rate [deg/s] : Outport  Port=12
  wires:
  Bus Selector/11 -> GPS alt [m]/1  "<Alt>"
  Bus Selector/10 -> GPS long [deg]/1  "<Long>"
  Bus Selector/9 -> GPS lat [deg]/1  "<Lat>"
  Bus Selector/8 -> Gain1/1  "<Yaw_rate>"
  Bus Selector/7 -> velocity [m/s]/1  "<Velocity>"
  Bus Selector/6 -> compas converter/1(rotz [rad]), Vector Concatenate1/3  "<OrientationYaw>"
  Bus Selector/5 -> Vector Concatenate1/2  "<OrientationPitch>"
  Bus Selector/4 -> Vector Concatenate1/1  "<OrientationRoll>"
  Vector Concatenate1/1 -> Gain/1
  Bus Selector/3 -> z [m]/1  "<PositionZ>"
  Bus Selector/2 -> y [m]/1  "<PositionY>"
  Bus Selector/1 -> x [m]/1  "<PositionX>"
  SELF/1 -> Bus Selector/1
  Gain/1 -> Demux2/1
  Demux2/1 -> rotx [deg]/1
  Demux2/2 -> roty [deg]/1
  Demux2/3 -> rotz [deg]/1
  compas converter/1(heading [deg]) -> heading [deg]/1
  Gain1/1 -> yaw rate [deg/s]/1

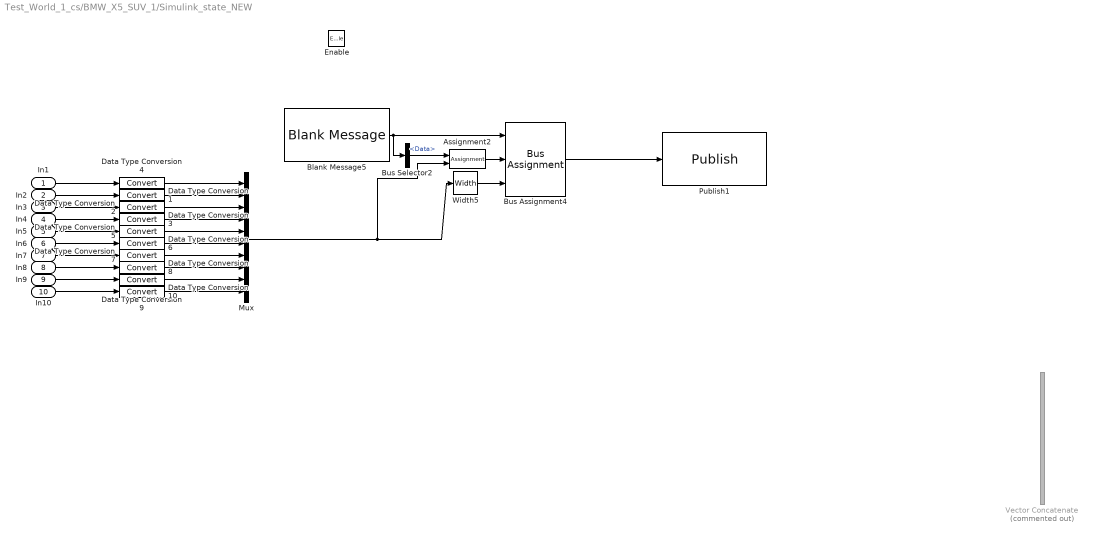
== system Test_World_1_cs/BMW_X5_SUV_1/Simulink_state_NEW ==
  In1 : Inport
  In2 : Inport  Port=2
  In3 : Inport  Port=3
  In4 : Inport  Port=4
  In5 : Inport  Port=5
  In6 : Inport  Port=6
  In7 : Inport  Port=7
  In8 : Inport  Port=8
  In9 : Inport  Port=9
  In10 : Inport  Port=10
  Enable : EnablePort
  Assignment2 : Assignment  OutputInitialize=Specify size for each dimension in table  DiagnosticForDimensions=Warning  IndexOptions=Starting index (dialog)  Indices=1  OutputSizes=1000
  Blank Message5 : robotlib/Blank Message  messageClass=Message  entityType=std_msgs/Int32MultiArray  messageType=std_msgs/Int32MultiArray  SampleTime=inf
      settings: SourceProductBaseCode=RO
  Bus Assignment4 : BusAssignment  AssignedSignals=Data,Data_SL_Info.CurrentLength
  Bus Selector2 : BusSelector  OutputSignals=Data
  Data Type Conversion{1..10} (10 alike) : DataTypeConversion
  Mux : Mux  Inputs=10
  Publish1 : robotlib/Publish  topicSource=Specify your own  topic=/Simulink_state  messageType=std_msgs/Int32MultiArray  messageQueueLength=1
      settings: SourceProductBaseCode=RO
  Vector Concatenate : Concatenate  Commented=on  NumInputs=10
  Width5 : Width  DataType=uint32
  wires:
  Assignment2/1 -> Bus Assignment4/2
  Blank Message5/1 -> Bus Assignment4/1, Bus Selector2/1
  Bus Selector2/1 -> Assignment2/1  "<Data>"
  In7/1 -> Data Type Conversion7/1
  In10/1 -> Data Type Conversion10/1
  In9/1 -> Data Type Conversion9/1
  In8/1 -> Data Type Conversion8/1
  In6/1 -> Data Type Conversion6/1
  In5/1 -> Data Type Conversion5/1
  In4/1 -> Data Type Conversion3/1
  In3/1 -> Data Type Conversion2/1
  In2/1 -> Data Type Conversion1/1
  Data Type Conversion10/1 -> Mux/10
  Data Type Conversion9/1 -> Mux/9
  Data Type Conversion8/1 -> Mux/8
  Data Type Conversion7/1 -> Mux/7
  Data Type Conversion6/1 -> Mux/6
  Data Type Conversion5/1 -> Mux/5
  Data Type Conversion3/1 -> Mux/4
  Data Type Conversion2/1 -> Mux/3
  Data Type Conversion1/1 -> Mux/2
  Width5/1 -> Bus Assignment4/3
  Mux/1 -> Width5/1, Assignment2/2
  Bus Assignment4/1 -> Publish1/1
  Data Type Conversion4/1 -> Mux/1
  In1/1 -> Data Type Conversion4/1

== system Test_World_1_cs/BMW_X5_SUV_1/Subsystem ==
  In1 : Inport
  In2 : Inport  Port=2
  In3 : Inport  Port=3
  In4 : Inport  Port=4
  In5 : Inport  Port=5
  Matrix Concatenate5 : Concatenate  NumInputs=4  Mode=Multidimensional array  ConcatenateDimension=2
  Reshape{1..4} (4 alike) : Reshape
  Rotate over Z : Subsystem
  Spherical to cartesian : Subsystem
  Out1 : Outport
  wires:
  In4/1 -> Reshape2/1
  In2/1 -> Reshape4/1
  Matrix Concatenate5/1 -> Out1/1
  Rotate over Z/1(Out1) -> Matrix Concatenate5/1
  Reshape3/1 -> Matrix Concatenate5/4
  Spherical to cartesian/3(Out3) -> Matrix Concatenate5/3
  Rotate over Z/2(Out2) -> Matrix Concatenate5/2
  In3/1 -> Reshape1/1
  Spherical to cartesian/2(Out2) -> Rotate over Z/3(In3)
  Reshape2/1 -> Spherical to cartesian/3(In3)
  Spherical to cartesian/1(Out1) -> Rotate over Z/2(In2)
  Reshape1/1 -> Spherical to cartesian/2(In2)
  In1/1 -> Rotate over Z/1(In1)
  Reshape4/1 -> Spherical to cartesian/1(In1)
  In5/1 -> Reshape3/1

== system Test_World_1_cs/BMW_X5_SUV_1/Subsystem1 ==
  In1 : Inport
  In2 : Inport  Port=2
  In3 : Inport  Port=3
  In4 : Inport  Port=4
  In5 : Inport  Port=5
  Matrix Concatenate5 : Concatenate  NumInputs=4  Mode=Multidimensional array  ConcatenateDimension=2
  Reshape{1..4} (4 alike) : Reshape
  Rotate over Z : Subsystem
  Spherical to cartesian : Subsystem
  Out1 : Outport
  wires:
  In4/1 -> Reshape2/1
  In2/1 -> Reshape4/1
  Matrix Concatenate5/1 -> Out1/1
  Rotate over Z/1(Out1) -> Matrix Concatenate5/1
  Reshape3/1 -> Matrix Concatenate5/4
  Spherical to cartesian/3(Out3) -> Matrix Concatenate5/3
  Rotate over Z/2(Out2) -> Matrix Concatenate5/2
  In3/1 -> Reshape1/1
  Spherical to cartesian/2(Out2) -> Rotate over Z/3(In3)
  Reshape2/1 -> Spherical to cartesian/3(In3)
  Spherical to cartesian/1(Out1) -> Rotate over Z/2(In2)
  Reshape1/1 -> Spherical to cartesian/2(In2)
  In1/1 -> Rotate over Z/1(In1)
  Reshape4/1 -> Spherical to cartesian/1(In1)
  In5/1 -> Reshape3/1

== system Test_World_1_cs/BMW_X5_SUV_1/Subsystem2 ==
  In1 : Inport
  In2 : Inport  Port=2
  In3 : Inport  Port=3
  In4 : Inport  Port=4
  In5 : Inport  Port=5
  Matrix Concatenate5 : Concatenate  NumInputs=4  Mode=Multidimensional array  ConcatenateDimension=2
  Reshape{1..4} (4 alike) : Reshape
  Rotate over Z : Subsystem
  Spherical to cartesian : Subsystem
  Out1 : Outport
  wires:
  In4/1 -> Reshape2/1
  In2/1 -> Reshape4/1
  Matrix Concatenate5/1 -> Out1/1
  Rotate over Z/1(Out1) -> Matrix Concatenate5/1
  Reshape3/1 -> Matrix Concatenate5/4
  Spherical to cartesian/3(Out3) -> Matrix Concatenate5/3
  Rotate over Z/2(Out2) -> Matrix Concatenate5/2
  In3/1 -> Reshape1/1
  Spherical to cartesian/2(Out2) -> Rotate over Z/3(In3)
  Reshape2/1 -> Spherical to cartesian/3(In3)
  Spherical to cartesian/1(Out1) -> Rotate over Z/2(In2)
  Reshape1/1 -> Spherical to cartesian/2(In2)
  In1/1 -> Rotate over Z/1(In1)
  Reshape4/1 -> Spherical to cartesian/1(In1)
  In5/1 -> Reshape3/1

== system Test_World_1_cs/BMW_X5_SUV_1/Subsystem3 ==
  In1 : Inport
  In2 : Inport  Port=2
  In3 : Inport  Port=3
  In4 : Inport  Port=4
  In5 : Inport  Port=5
  Matrix Concatenate5 : Concatenate  NumInputs=4  Mode=Multidimensional array  ConcatenateDimension=2
  Reshape{1..4} (4 alike) : Reshape
  Rotate over Z : Subsystem
  Spherical to cartesian : Subsystem
  Out1 : Outport
  wires:
  In4/1 -> Reshape2/1
  In2/1 -> Reshape4/1
  Matrix Concatenate5/1 -> Out1/1
  Rotate over Z/1(Out1) -> Matrix Concatenate5/1
  Reshape3/1 -> Matrix Concatenate5/4
  Spherical to cartesian/3(Out3) -> Matrix Concatenate5/3
  Rotate over Z/2(Out2) -> Matrix Concatenate5/2
  In3/1 -> Reshape1/1
  Spherical to cartesian/2(Out2) -> Rotate over Z/3(In3)
  Reshape2/1 -> Spherical to cartesian/3(In3)
  Spherical to cartesian/1(Out1) -> Rotate over Z/2(In2)
  Reshape1/1 -> Spherical to cartesian/2(In2)
  In1/1 -> Rotate over Z/1(In1)
  Reshape4/1 -> Spherical to cartesian/1(In1)
  In5/1 -> Reshape3/1

== system Test_World_1_cs/BMW_X5_SUV_1/Subsystem4 ==
  Enable : EnablePort
  Bus Selector : BusSelector  OutputSignals=Pose.Position.X
  Subscribe : robotlib/Subscribe  topicSource=Specify your own  topic=/current_pose  messageType=geometry_msgs/PoseStamped  sampleTime=-1  messageQueueLength=1
      settings: SourceProductBaseCode=RO
  Terminator_6 : Terminator
  To Workspace : ToWorkspace  VariableName=Values_of_X  SaveFormat=Timeseries  SampleTime=-1
  wires:
  Subscribe/1 -> Terminator_6/1
  Subscribe/2 -> Bus Selector/1
  Bus Selector/1 -> To Workspace/1  "<X>"

== system Test_World_1_cs/BMW_X5_SUV_1/camera_CM_Demux ==
  In1 : Inport
  Selector : Selector  NumberOfDimensions=2  InputPortWidth=3  IndexOptions=Index vector (dialog),Index vector (dialog)  Indices=-1,1:hres  OutputSizes=1,1
  Selector1 : Selector  NumberOfDimensions=2  InputPortWidth=3  IndexOptions=Index vector (dialog),Index vector (dialog)  Indices=-1,hres+1:hres*2  OutputSizes=1,1
  Selector2 : Selector  NumberOfDimensions=2  InputPortWidth=3  IndexOptions=Index vector (dialog),Index vector (dialog)  Indices=-1,hres*2+1:hres*3  OutputSizes=1,1
  R : Outport
  G : Outport  Port=2
  B : Outport  Port=3
  wires:
  In1/1 -> Selector1/1, Selector/1, Selector2/1
  Selector/1 -> R/1
  Selector1/1 -> G/1
  Selector2/1 -> B/1
